simulink model "ForceController"  (R2017a)
settings: Solver=FixedStepDiscrete  StartTime=0.0  StopTime=10.0  FixedStep=0.002  RelTol=1e-3
values from neighbouring files (symbols this model uses):
  D = 0.0    [param.sldd]
  filter_den : value not decoded    [param.sldd]
  filter_num : value not decoded    [param.sldd]
  I = 1.0    [param.sldd]
  K_lamuda = 0.02    [param.sldd]
  N = 0.0    [param.sldd]
  P = 10.0    [param.sldd]
  saturation_lower_limit = -100.0    [param.sldd]
  saturation_upper_limit = 100.0    [param.sldd]
libraries: dspfdesign x6, simulink x2
settings Model: DataDictionary=param.sldd  ModifiedByFormat=The MathWorks Inc.  Creator=The MathWorks, Inc.  LastModifiedBy=The MathWorks Inc.
settings DataIOCC: SaveFormat=Array  SaveOutput=off  SignalLogging=off  DSMLogging=off  SaveTime=off
settings OptimizationCC: ExpressionDepthLimit=2147483647  ZeroExternalMemoryAtStartup=off  EfficientFloat2IntCast=on
settings DebuggingCC: SolverPrmCheckMsg=warning  ParameterTunabilityLossMsg=error  FcnCallInpInsideContextMsg=warning  UniqueDataStoreMsg=error  AssertControl=DisableAll  AllowSymbolicDim=off  StateNameClashWarn=warning  StrictBusMsg=ErrorOnBusTreatedAsVector  SFUnexpectedBacktrackingDiag=warning  SFNoUnconditionalDefaultTransitionDiag=warning  SFExecutionAtInitializationDiag=none
settings HardwareCC: ProdBitPerPointer=32  ProdBitPerSizeT=32  ProdBitPerPtrDiffT=32  ProdLargestAtomicFloat=None  ProdIntDivRoundTo=Undefined  ProdEndianess=Unspecified  ProdWordSize=32  ProdHWDeviceType=32-bit Generic
settings ModelReferenceCC: PropagateSignalLabelsOutOfModel=off
settings SFSimCC: MATLABDynamicMemAlloc=off
settings RTWCC: SystemTargetFile=ert.tlc  GenCodeOnly=on  PackageName=ForceController  TemplateMakefile=ert_default_tmf  Description=Embedded Coder  GenerateReport=on  IncludeHyperlinkInReport=on  LaunchReport=on  TargetLang=C++  GenerateTraceInfo=on  GenerateTraceReport=on  GenerateTraceReportSl=on  GenerateTraceReportSf=on  GenerateTraceReportEml=on  GenerateWebview=on  GenerateCodeMetricsReport=on
settings CodeAppCC: ForceParamTrailComments=on  OperatorAnnotations=on  SimulinkDataObjDesc=on  SFDataObjDesc=on  MATLABFcnDesc=on  InsertBlockDesc=on  MATLABSourceComments=on
settings ERTTargetCC: TargetLangStandard=C++03 (ISO)  MultiwordLength=2048  GenerateSampleERTMain=on  SuppressErrorStatus=on  MultiInstanceERTCode=on  CodeInterfacePackaging=C++ class  SupportComplex=off  MultiInstanceErrorCode=Warning  RootIOFormat=Structure reference  ERTCustomFileTemplate=example_file_process.tlc  ERTFilePackagingFormat=Compact
settings ConfigComp: CovMetricSettings=dw  CovHtmlReporting=on  CovSaveCumulativeToWorkspaceVar=on  CovSaveSingleToWorkspaceVar=on  CovExternalEMLEnable=off  CovSFcnEnable=off

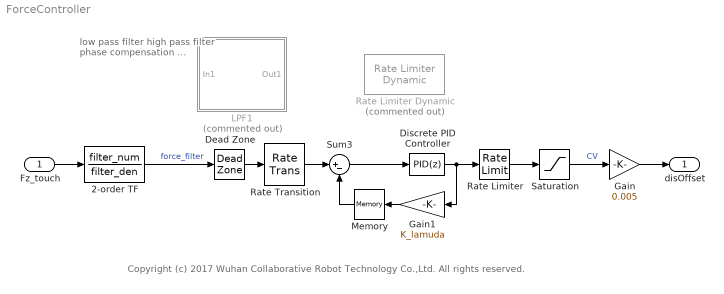
== system ForceController ==
  note: Copyright (c) 2017 Wuhan Collaborative Robot Technology Co.,Ltd. All rights reserved.
  note: low pass filter
      | high pass filter
      | phase compensation
      | ...
  Fz_touch : Inport  OutDataTypeStr=double  PortDimensions=1
  2-order TF : DiscreteTransferFcn  Numerator=filter_num  Denominator=filter_den
  Dead Zone : DeadZone  LowerValue=dead_zone_start  UpperValue=dead_zone_end  SaturateOnIntegerOverflow=on
  Discrete PID Controller : simulink/Continuous/PID Controller  Controller=PID  TimeDomain=Discrete-time  SampleTime=0.008  IntegratorMethod=Forward Euler  FilterMethod=Forward Euler  Form=Parallel  UseFilter=on  ControllerParametersSource=internal  P=P  I=I  D=D  N=N  InitialConditionSource=internal  InitialConditionForIntegrator=0  InitialConditionForFilter=0  ExternalReset=none  LimitOutput=off  UpperSaturationLimit=inf  LowerSaturationLimit=-inf  LinearizeAsGain=off  AntiWindupMode=none  Kb=1  TrackingMode=off  Kt=1  PParamMin=[]  PParamMax=[]  PParamDataTypeStr=double  IParamMin=[]  IParamMax=[]  IParamDataTypeStr=double  DParamMin=[]  DParamMax=[]  DParamDataTypeStr=double  NParamMin=[]  NParamMax=[]  NParamDataTypeStr=double  KbParamMin=[]  KbParamMax=[]  KtParamMin=[]  KtParamMax=[]  POutMin=[]  POutMax=[]  IOutMin=[]  IOutMax=[]  DOutMin=[]  DOutMax=[]  NOutMin=[]  NOutMax=[]  KbOutMin=[]  KbOutMax=[]  KtOutMin=[]  KtOutMax=[]  IntegratorOutMin=[]  IntegratorOutMax=[]  FilterOutMin=[]  FilterOutMax=[]  SumOutMin=[]  SumOutMax=[]  SumI1OutMin=[]  SumI1OutMax=[]  SumI2OutMin=[]  SumI2OutMax=[]  SumI3OutMin=[]  SumI3OutMax=[]  SumDOutMin=[]  SumDOutMax=[]  SaturationOutMin=[]  SaturationOutMax=[]  IntegratorContinuousStateAttributes=''  IntegratorStateMustResolveToSignalObject=off  IntegratorRTWStateStorageClass=Auto  FilterContinuousStateAttributes=''  FilterStateMustResolveToSignalObject=off  FilterRTWStateStorageClass=Auto  DifferentiatorICPrevScaledInput=0  DifferentiatorOutMin=[]  DifferentiatorOutMax=[]  InitialConditionSetting=State (most efficient)
  Gain : Gain  Gain=0.005
  Gain1 : Gain  Gain=K_lamuda
  LPF1 : Subsystem  Commented=on
  Memory : Memory
  Rate Limiter : RateLimiter  RisingSlewLimit=1000  FallingSlewLimit=-1000  SampleTimeMode=inherited
  Rate Limiter Dynamic : simulink/Discontinuities/Rate Limiter Dynamic  Commented=on
      settings: SourceProductName=Simulink
  Rate Transition : RateTransition
  Saturation : Saturate  UpperLimit=saturation_upper_limit  LowerLimit=saturation_lower_limit
  Sum3 : Sum  Inputs=|+-
  disOffset : Outport  OutDataTypeStr=double  PortDimensions=1
  wires:
  Rate Limiter/1 -> Saturation/1
  Dead Zone/1 -> Rate Transition/1
  2-order TF/1 -> Dead Zone/1  "force_filter"
  Fz_touch/1 -> 2-order TF/1
  Saturation/1 -> Gain/1  "CV"
  Rate Transition/1 -> Sum3/1
  Discrete PID Controller/1 -> Rate Limiter/1, Gain1/1
  Sum3/1 -> Discrete PID Controller/1
  Gain1/1 -> Memory/1
  Gain/1 -> disOffset/1
  Memory/1 -> Sum3/2

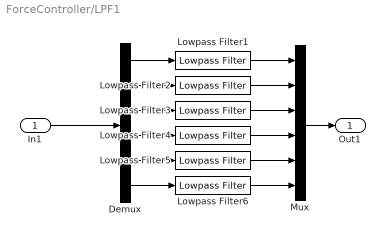
== system ForceController/LPF1 ==
  In1 : Inport
  Demux : Demux  Outputs=6
  Lowpass Filter{1..6} (6 alike) : dspfdesign/Lowpass Filter  FilterType=IIR  DesignForMinimumOrder=on  FilterOrder=50  PassbandFrequency=10  StopbandFrequency=40  PassbandRipple=2  StopbandAttenuation=20  InheritSampleRate=off  SampleRate=500  SimulateUsing=Interpreted execution  roundingMode=Floor  coeffsDataTypeStr=fixdt(1,16)
  Mux : Mux  Inputs=6
  Out1 : Outport
  wires:
  Mux/1 -> Out1/1
  Demux/6 -> Lowpass Filter6/1
  Demux/5 -> Lowpass Filter5/1
  Demux/1 -> Lowpass Filter1/1
  Demux/2 -> Lowpass Filter2/1
  In1/1 -> Demux/1
  Demux/4 -> Lowpass Filter4/1
  Lowpass Filter5/1 -> Mux/5
  Lowpass Filter3/1 -> Mux/3
  Lowpass Filter2/1 -> Mux/2
  Lowpass Filter6/1 -> Mux/6
  Demux/3 -> Lowpass Filter3/1
  Lowpass Filter1/1 -> Mux/1
  Lowpass Filter4/1 -> Mux/4
